simulink model "motor_control_of_a_drone"  (R2022a)
settings: Solver=VariableStepAuto  StartTime=0.0  StopTime=15  RelTol=1e-3
libraries: spsMosfetLib x6, spsSeriesRLCBranchLib x3, spsVoltageMeasurementLib x3, spsDCVoltageSourceLib x1, spspowerguiLib x1
settings Model: Creator=siddh  LastModifiedBy=siddh

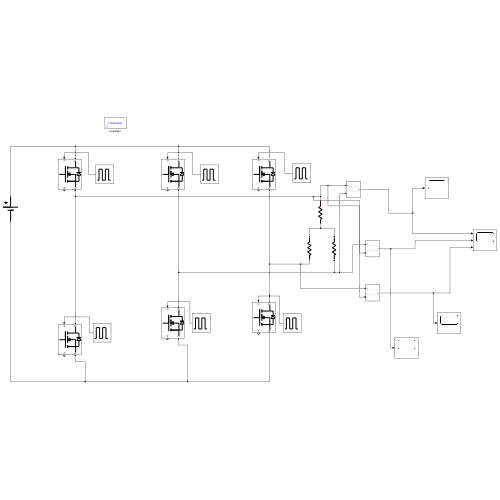
[thumbnail: Simulink's stored preview of the top-level diagram]
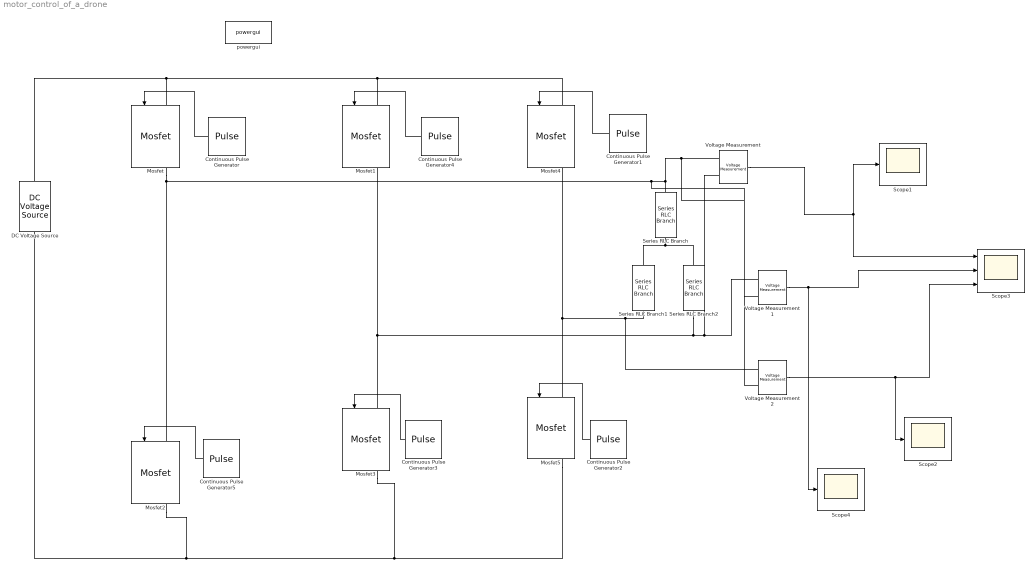
== system motor_control_of_a_drone ==
  Continuous Pulse Generator : DiscretePulseGenerator  PulseType=Time based  Period=6  PulseWidth=100/3
  Continuous Pulse Generator1 : DiscretePulseGenerator  PulseType=Time based  Period=6  PulseWidth=100/3  PhaseDelay=4
  Continuous Pulse Generator2 : DiscretePulseGenerator  PulseType=Time based  Period=6  PulseWidth=100/3  PhaseDelay=1
  Continuous Pulse Generator3 : DiscretePulseGenerator  PulseType=Time based  Period=6  PulseWidth=100/3  PhaseDelay=-1
  Continuous Pulse Generator4 : DiscretePulseGenerator  PulseType=Time based  Period=6  PulseWidth=100/3  PhaseDelay=2
  Continuous Pulse Generator5 : DiscretePulseGenerator  PulseType=Time based  Period=6  PulseWidth=100/3  PhaseDelay=3
  DC Voltage Source : spsDCVoltageSourceLib/DC Voltage Source  Amplitude=10  Measurements=None
  Mosfet{,1..5} (6 alike) : spsMosfetLib/Mosfet  Ron=0.1  Lon=0  Rd=0.01  Vfd=0  IC=0  Rs=1e5  Cs=inf  Measurements=on
  Scope1 : Scope
  Scope2 : Scope
  Scope3 : Scope  NumInputPorts=3
  Scope4 : Scope
  Series RLC Branch : spsSeriesRLCBranchLib/Series RLC Branch  LConnTagsString=__new0  RConnTagsString=__new0  BranchType=R  Resistance=10  Inductance=1e-3  SetiL0=off  InitialCurrent=0  Capacitance=1e-6  Setx0=off  InitialVoltage=0  Measurements=None
  Series RLC Branch1 : spsSeriesRLCBranchLib/Series RLC Branch  LConnTagsString=__new0  RConnTagsString=__new0  BranchType=R  Resistance=10  Inductance=1e-3  SetiL0=off  InitialCurrent=0  Capacitance=1e-6  Setx0=off  InitialVoltage=0  Measurements=None
  Series RLC Branch2 : spsSeriesRLCBranchLib/Series RLC Branch  LConnTagsString=__new0  RConnTagsString=__new0  BranchType=R  Resistance=10  Inductance=1e-3  SetiL0=off  InitialCurrent=0  Capacitance=1e-6  Setx0=off  InitialVoltage=0  Measurements=None
  Voltage Measurement : spsVoltageMeasurementLib/Voltage Measurement  PhasorSimulation=off  OutputType=Complex  PSBequivalent=0
  Voltage Measurement1 : spsVoltageMeasurementLib/Voltage Measurement  PhasorSimulation=off  OutputType=Complex  PSBequivalent=0
  Voltage Measurement2 : spsVoltageMeasurementLib/Voltage Measurement  PhasorSimulation=off  OutputType=Complex  PSBequivalent=0
  powergui : spspowerguiLib/powergui  Priority=1  SimulationMode=Continuous  SampleTime=50e-6  frequency=60  Iterations=50  frequencyindice=0  Pbase=100e6  ErrMax=1e-4  UnitsV=kV  UnitsW=MW  buscounter=0  FunctionMessages=off  echomessages=off  EnableUseOfTLC=off  CurrentSourceSwitches=off  DisableSnubberDevices=off  DisableRonSwitches=off  DisableVfSwitches=off  DisplayEquations=off  AutomaticDiscreteSolvers=off  SolverType=Tustin/Backward Euler (TBE)  Interpol=off  ExternalGateDelay=off  methode=off  Ts=100  x0status=blocks  SPID=on  SwTol=0  HookPort=off  NonlinearTolerance=1e-4  nMaxIteration=100  ContinueOnMaxIteration=off  RestoreLinks=warning  ResistiveCurrentMeasurement=off  Frange=[0:2:500]  Ylog=off  Xlog=on  ShowGrid=off  save=off  variable=ZData  structure=0  ZoomFFT=off  StartTime=0.0  cycles=1  DisplayStyle=1  fundamental=60  FreqAxis=off  MaxFrequency=1000  frequencyindicesteady=1  RmsSteady=1  display=off
  wires:
  Continuous Pulse Generator/1 -> Mosfet/1
  Continuous Pulse Generator2/1 -> Mosfet5/1
  Continuous Pulse Generator3/1 -> Mosfet3/1
  Continuous Pulse Generator4/1 -> Mosfet1/1
  Continuous Pulse Generator1/1 -> Mosfet4/1
  Continuous Pulse Generator5/1 -> Mosfet2/1
  Voltage Measurement/1 -> Scope1/1, Scope3/1
  Voltage Measurement1/1 -> Scope4/1, Scope3/2
  Voltage Measurement2/1 -> Scope2/1, Scope3/3
  connections:
  DC Voltage Source/RConn1 -- Mosfet4/LConn1 -- Mosfet1/LConn1 -- Mosfet/LConn1
  Mosfet/RConn1 -- Voltage Measurement2/LConn2 -- Voltage Measurement1/LConn2 -- Voltage Measurement/LConn1 -- Series RLC Branch/LConn1 -- Mosfet2/LConn1
  Mosfet2/RConn1 -- Mosfet3/RConn1 -- Mosfet5/RConn1 -- DC Voltage Source/LConn1
  Mosfet3/LConn1 -- Voltage Measurement/LConn2 -- Voltage Measurement1/LConn1 -- Series RLC Branch2/RConn1 -- Mosfet1/RConn1
  Mosfet5/LConn1 -- Voltage Measurement2/LConn1 -- Series RLC Branch1/RConn1 -- Mosfet4/RConn1
  Series RLC Branch1/LConn1 -- Series RLC Branch2/LConn1 -- Series RLC Branch/RConn1
